simulink model "WEEK1_QN2"  (R2020b)
settings: Solver=VariableStepAuto  StartTime=0.0  StopTime=10.0  RelTol=1e-3
model workspace (MAT data in the model file):
  b = 300
  k1 = 6000
  k2 = 150000
  m1 = 500
  m2 = 50
settings Model: Creator=dell  LastModifiedBy=dell

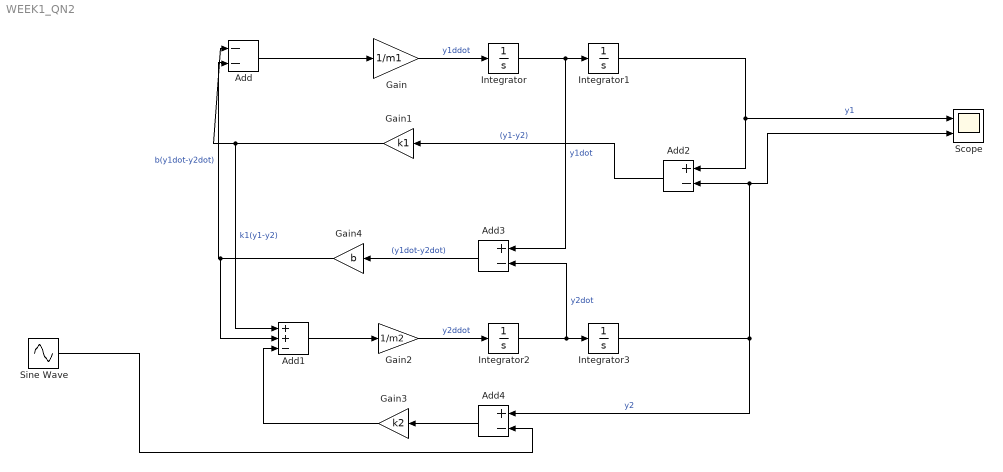
== system WEEK1_QN2 ==
  Add : Sum  Inputs=--
  Add1 : Sum  Inputs=++-
  Add2 : Sum  Inputs=+-
  Add3 : Sum  Inputs=+-
  Add4 : Sum  Inputs=+-
  Gain : Gain  Gain=1/m1
  Gain1 : Gain  Gain=k1
  Gain2 : Gain  Gain=1/m2
  Gain3 : Gain  Gain=k2
  Gain4 : Gain  Gain=b
  Integrator{,1..3} (4 alike) : Integrator
  Scope : Scope  NumInputPorts=2
  Sine Wave : Sin  SampleTime=0
  wires:
  Gain/1 -> Integrator/1  "y1ddot"
  Integrator/1 -> Add3/1, Integrator1/1  "y1dot"
  Gain2/1 -> Integrator2/1  "y2ddot"
  Integrator2/1 -> Add3/2, Integrator3/1  "y2dot"
  Integrator1/1 -> Scope/1, Add2/1  "y1"
  Integrator3/1 -> Add4/1, Scope/2, Add2/2  "y2"
  Add3/1 -> Gain4/1  "(y1dot-y2dot)"
  Add2/1 -> Gain1/1  "(y1-y2)"
  Gain1/1 -> Add1/1, Add/1  "k1(y1-y2)"
  Gain4/1 -> Add1/2, Add/2  "b(y1dot-y2dot)"
  Add1/1 -> Gain2/1
  Add/1 -> Gain/1
  Sine Wave/1 -> Add4/2
  Add4/1 -> Gain3/1
  Gain3/1 -> Add1/3
